simulink model "TemperatureSensor"  (R2020b)
settings: Solver=VariableStepAuto  StartTime=0.0  StopTime=10.0  RelTol=1e-3
settings Model: Creator=99003778  LastModifiedBy=99003778

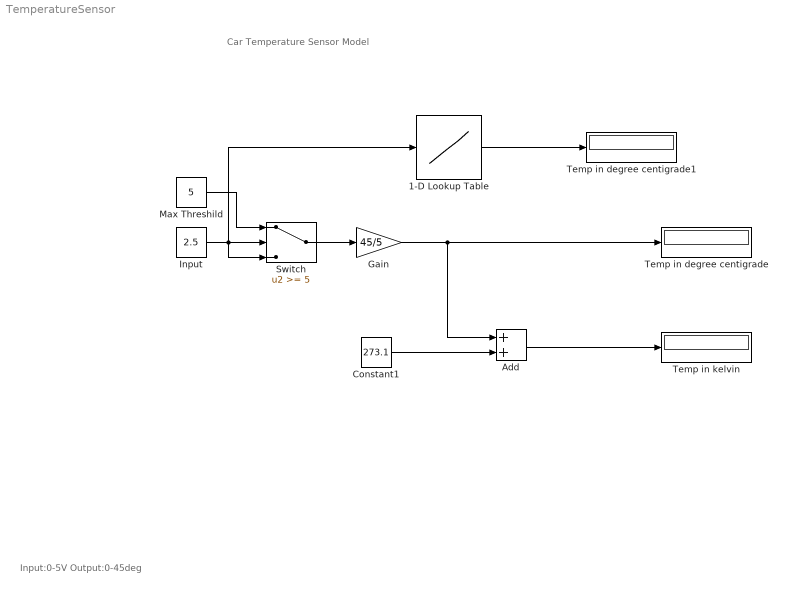
== system TemperatureSensor ==
  note: Input:0-5V
      | Output:0-45deg
  note: Car Temperature Sensor Model
  1-D Lookup Table : Lookup_n-D  NumberOfTableDimensions=1  BreakpointsForDimension1=[0:0.1:5]  Table=[0:0.9:45]  ExtrapMethod=Clip  InternalRulePriority=Speed  RndMeth=Simplest  InputSameDT=on
  Add : Sum
  Constant1 : Constant  Value=273.1
  Gain : Gain  Gain=45/5
  Input : Constant  Value=2.5  VectorParams1D=off
  Max Threshild : Constant  Value=5
  Switch : Switch  Threshold=5
  Temp in degree centigrade : Display
  Temp in degree centigrade1 : Display
  Temp in kelvin : Display
  wires:
  Gain/1 -> Add/1, Temp in degree centigrade/1
  Constant1/1 -> Add/2
  Add/1 -> Temp in kelvin/1
  Input/1 -> 1-D Lookup Table/1, Switch/3, Switch/2
  Switch/1 -> Gain/1
  Max Threshild/1 -> Switch/1
  1-D Lookup Table/1 -> Temp in degree centigrade1/1
